simulink model "B5B3"  (R2015a)
settings: Solver=ode45  StartTime=0.0  StopTime=10.0  RelTol=1e-3
libraries: dspsrcs4 x4, commfilt2 x2, commchan3 x1, commsink2 x1, commutil2 x1, commrandsrc2 x1, dspstat3 x1
settings Model: Creator=Ekko  LastModifiedBy=Ekko

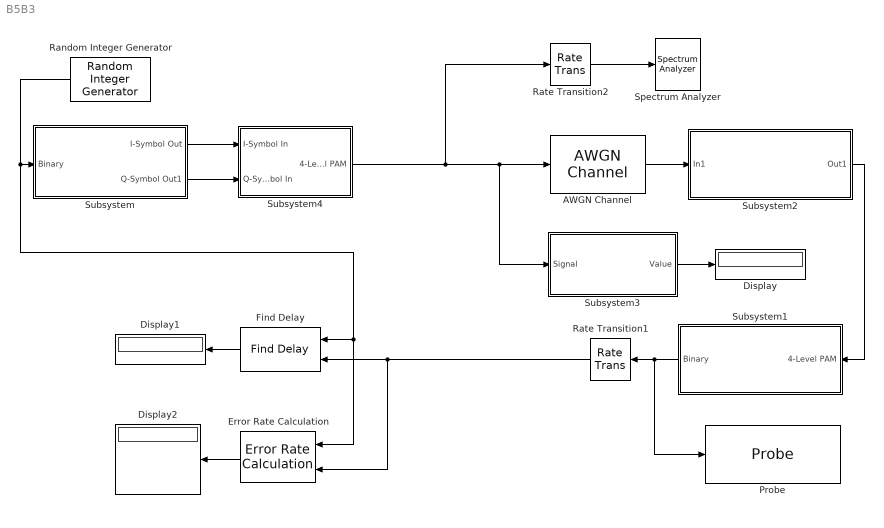
== system B5B3 ==
  AWGN Channel : commchan3/AWGN Channel  InputProcessing=Columns as channels (frame based)  seed=67  noiseMode="Signal to noise ratio  (Eb/No)"  EbNodB=8  EsNodB=10  SNRdB=10  bitsPerSym=1  Ps=1  Tsym=1  variance=1
  Display : Display
  Display1 : Display
  Display2 : Display
  Error Rate Calculation : commsink2/Error Rate Calculation  N=0  st_delay=0  cp_mode=Entire frame  subframe=[]  PMode=Port  WsName=ErrorVec  RsMode2=off  stop=off  numErr=100  maxBits=1e6
  Find Delay : commutil2/Find Delay  corrLength=200  chgSigOP=off  stopUpdate=off  numConstDelay=3
  Probe : Probe  ProbeWidth=off  ProbeComplexSignal=off  ProbeSignalDimensions=on
  Random Integer Generator : commrandsrc2/Random Integer Generator  mul=2  seed=37  Ts=1e-5  frameBased=off  sampPerFrame=1  orient=off  outDataType=double
  Rate Transition1 : RateTransition  OutPortSampleTime=1e-5
  Rate Transition2 : RateTransition  OutPortSampleTime=1e-5
  Spectrum Analyzer : SpectrumAnalyzer
  Subsystem : Subsystem
  Subsystem1 : Subsystem
  Subsystem2 : Subsystem
  Subsystem3 : Subsystem
  Subsystem4 : Subsystem
  wires:
  AWGN Channel/1 -> Subsystem2/1(In1)
  Subsystem1/1("Binary ") -> Probe/1, Rate Transition1/1
  Subsystem2/1(Out1) -> Subsystem1/1("4-Level PAM ")
  Subsystem3/1("Value ") -> Display/1
  Find Delay/1 -> Display1/1
  Error Rate Calculation/1 -> Display2/1
  Rate Transition1/1 -> Error Rate Calculation/2, Find Delay/2
  Subsystem/1(I-Symbol Out) -> Subsystem4/1(I-Symbol In)
  Subsystem/2(Q-Symbol Out1) -> Subsystem4/2(Q-Symbol In)
  Subsystem4/1(4-Level PAM) -> Rate Transition2/1, Subsystem3/1("Signal "), AWGN Channel/1
  Random Integer Generator/1 -> Find Delay/1, Error Rate Calculation/1, Subsystem/1("Binary ")
  Rate Transition2/1 -> Spectrum Analyzer/1

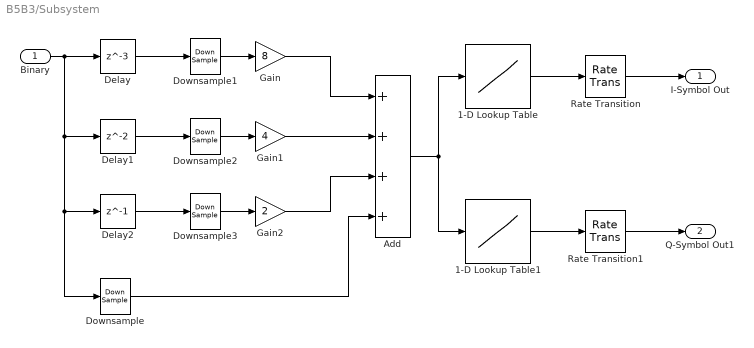
== system B5B3/Subsystem ==
  "Binary " : Inport
  1-D Lookup Table : Lookup_n-D  NumberOfTableDimensions=1  BreakpointsForDimension1=[0 1 2 3 4 5 6 7 8 9 10 11 12 13 14 15]  Table=[-1 -3 -1 -3 1 3 1 3 -1 -3 -1 -3 1 3 1 3]  InternalRulePriority=Speed  RndMeth=Simplest  InputSameDT=on
  1-D Lookup Table1 : Lookup_n-D  NumberOfTableDimensions=1  BreakpointsForDimension1=[0 1 2 3 4 5 6 7 8 9 10 11 12 13 14 15]  Table=[1 1 3 3 1 1 3 3 -1 -1 -3 -3 -1 -1 -3 -3]  InternalRulePriority=Speed  RndMeth=Simplest  InputSameDT=on
  Add : Sum  Inputs=4
  Delay : Delay  DelayLength=3
  Delay1 : Delay
  Delay2 : Delay  DelayLength=1
  Downsample{,1..3} (4 alike) : DownSample  N=4  RateOptions=Allow multirate processing
  Gain : Gain  Gain=8
  Gain1 : Gain  Gain=4
  Gain2 : Gain  Gain=2
  Rate Transition : RateTransition  OutPortSampleTime=1e-5
  Rate Transition1 : RateTransition  OutPortSampleTime=1e-5
  I-Symbol Out : Outport
  Q-Symbol Out1 : Outport  Port=2
  wires:
  "Binary "/1 -> Delay2/1, Downsample/1, Delay1/1, Delay/1
  Delay2/1 -> Downsample3/1
  Delay1/1 -> Downsample2/1
  Delay/1 -> Downsample1/1
  Downsample1/1 -> Gain/1
  Downsample2/1 -> Gain1/1
  Downsample3/1 -> Gain2/1
  Gain1/1 -> Add/2
  Gain/1 -> Add/1
  Gain2/1 -> Add/3
  Downsample/1 -> Add/4
  1-D Lookup Table1/1 -> Rate Transition1/1
  1-D Lookup Table/1 -> Rate Transition/1
  Add/1 -> 1-D Lookup Table1/1, 1-D Lookup Table/1
  Rate Transition1/1 -> Q-Symbol Out1/1
  Rate Transition/1 -> I-Symbol Out/1

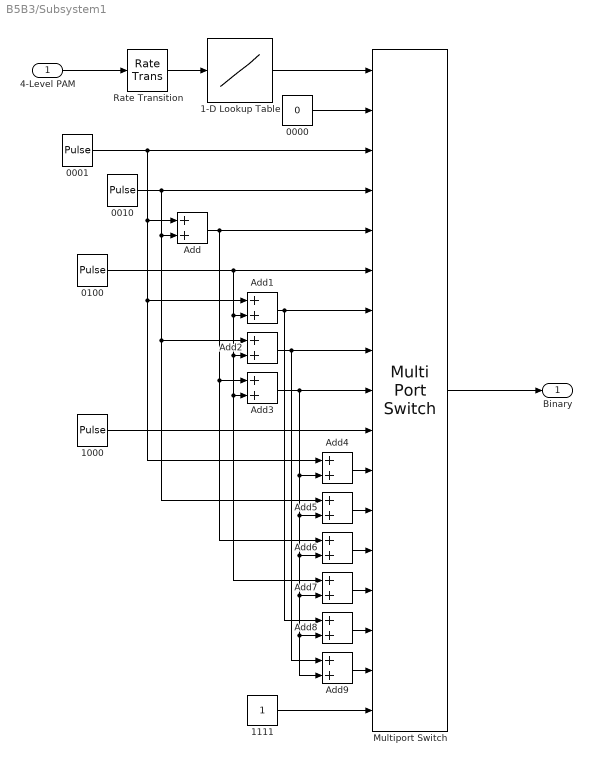
== system B5B3/Subsystem1 ==
  "4-Level PAM " : Inport
  0000 : Constant  Value=0  SampleTime=2e-5
  "0001 " : DiscretePulseGenerator  Amplitude=2  Period=50  PulseWidth=5  SampleTime=1e-5
  0010 : DiscretePulseGenerator  Amplitude=2  Period=10  PulseWidth=5  SampleTime=1e-5
  0100 : DiscretePulseGenerator  Amplitude=2  Period=10  PulseWidth=5  SampleTime=1e-5
  1-D Lookup Table : Lookup_n-D  NumberOfTableDimensions=1  BreakpointsForDimension1=[0 1]  Table=[-5 5]  InternalRulePriority=Speed  RndMeth=Simplest  InputSameDT=on
  1000 : DiscretePulseGenerator  Amplitude=2  Period=10  PulseWidth=5  SampleTime=1e-5
  "1111 " : Constant  SampleTime=2e-5
  Add{,1..9} (10 alike) : Sum
  Multiport Switch : MultiPortSwitch  Inputs=16  DiagnosticForDefault=None
  Rate Transition : RateTransition  OutPortSampleTime=1e-5
  "Binary " : Outport
  wires:
  Rate Transition/1 -> 1-D Lookup Table/1
  "4-Level PAM "/1 -> Rate Transition/1
  1-D Lookup Table/1 -> Multiport Switch/1
  0010/1 -> Add/2, Add2/1, Add5/1, Multiport Switch/4
  Multiport Switch/1 -> "Binary "/1
  "0001 "/1 -> Add/1, Add1/1, Add4/1, Multiport Switch/3
  0000/1 -> Multiport Switch/2
  "1111 "/1 -> Multiport Switch/17
  0100/1 -> Add1/2, Add2/2, Add3/2, Add7/1, Multiport Switch/6
  Add/1 -> Add6/1, Add3/1, Multiport Switch/5
  1000/1 -> Multiport Switch/10
  Add3/1 -> Add4/2, Add5/2, Add6/2, Add7/2, Add8/2, Add9/2, Multiport Switch/9
  Add2/1 -> Add9/1, Multiport Switch/8
  Add1/1 -> Add8/1, Multiport Switch/7
  Add4/1 -> Multiport Switch/11
  Add5/1 -> Multiport Switch/12
  Add6/1 -> Multiport Switch/13
  Add7/1 -> Multiport Switch/14
  Add8/1 -> Multiport Switch/15
  Add9/1 -> Multiport Switch/16

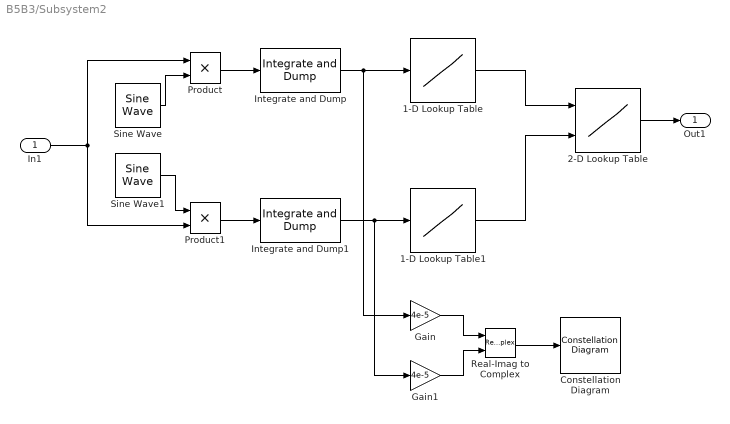
== system B5B3/Subsystem2 ==
  In1 : Inport
  1-D Lookup Table : Lookup_n-D  NumberOfTableDimensions=1  BreakpointsForDimension1=[0 1]  Table=[-5 5]  InternalRulePriority=Speed  RndMeth=Simplest  InputSameDT=on
  1-D Lookup Table1 : Lookup_n-D  NumberOfTableDimensions=1  BreakpointsForDimension1=[0 1]  Table=[-5 5]  InternalRulePriority=Speed  RndMeth=Simplest  InputSameDT=on
  2-D Lookup Table : Lookup_n-D  BreakpointsForDimension1=[1:3]  BreakpointsForDimension2=[1:3]  InternalRulePriority=Speed  RndMeth=Simplest  InputSameDT=on
  Constellation Diagram : ConstellationDiagram
  Gain : Gain  Gain=4e-5
  Gain1 : Gain  Gain=4e-5
  Integrate and Dump : commfilt2/Integrate and Dump  obssamples=8  offsetsamples=0  nodump=off  roundingMode=Floor  overflowMode=off
  Integrate and Dump1 : commfilt2/Integrate and Dump  obssamples=8  offsetsamples=0  nodump=off  roundingMode=Floor  overflowMode=off
  Product : Product
  Product1 : Product
  Real-Imag to Complex : RealImagToComplex
  Sine Wave : dspsrcs4/Sine Wave  Amplitude=1  Frequency=2000  Phase=0  SampleMode=Discrete  OutComplex=Real  CompMethod=Trigonometric fcn  TableSize=Speed  SampleTime=2e-5  SamplesPerFrame=1  ResetState=Restart at time zero  dataType=double  wordLen=16  udDataType=sfix(16)  fracBitsMode=Best precision  numFracBits=15  OutDataTypeStr=double  LastOutDataTypeStr=double
  Sine Wave1 : dspsrcs4/Sine Wave  Amplitude=1  Frequency=4000  Phase=0  SampleMode=Discrete  OutComplex=Real  CompMethod=Trigonometric fcn  TableSize=Speed  SampleTime=2e-5  SamplesPerFrame=1  ResetState=Restart at time zero  dataType=double  wordLen=16  udDataType=sfix(16)  fracBitsMode=Best precision  numFracBits=15  OutDataTypeStr=double  LastOutDataTypeStr=double
  Out1 : Outport
  wires:
  Product1/1 -> Integrate and Dump1/1
  Product/1 -> Integrate and Dump/1
  Sine Wave/1 -> Product/2
  In1/1 -> Product1/2, Product/1
  Sine Wave1/1 -> Product1/1
  Integrate and Dump/1 -> Gain/1, 1-D Lookup Table/1
  Integrate and Dump1/1 -> Gain1/1, 1-D Lookup Table1/1
  1-D Lookup Table/1 -> 2-D Lookup Table/1
  2-D Lookup Table/1 -> Out1/1
  Gain/1 -> Real-Imag to Complex/1
  Gain1/1 -> Real-Imag to Complex/2
  Real-Imag to Complex/1 -> Constellation Diagram/1
  1-D Lookup Table1/1 -> 2-D Lookup Table/2

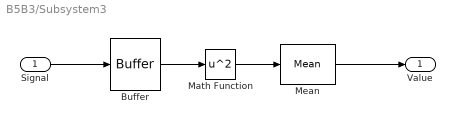
== system B5B3/Subsystem3 ==
  "Signal " : Inport
  Buffer : Buffer  TreatMby1Signals=One channel
  Math Function : Math  Operator=square  SaturateOnIntegerOverflow=on
  Mean : dspstat3/Mean  run=off  reset_popup=None  InputProcessing=Columns as channels (frame based)  directionMode=Each column  dimension=1  treatSBRowAsCol=off  roiEnable=off  roiType=Rectangles  roiPortion=Entire ROI  roiOutput=Individual statistics for each ROI  roiFlag=off  outputDataTypeStr=Inherit: Same as accumulator  outputLastDataTypeStr=Inherit: Same as accumulator  outputMin=[]  outputMax=[]  roundingMode=Floor  overflowMode=off
  "Value " : Outport
  wires:
  "Signal "/1 -> Buffer/1
  Mean/1 -> "Value "/1
  Math Function/1 -> Mean/1
  Buffer/1 -> Math Function/1

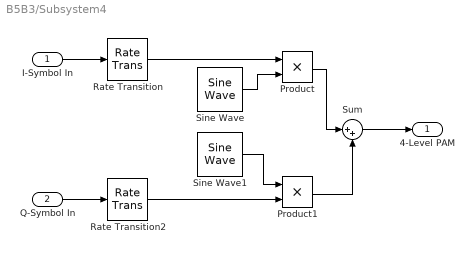
== system B5B3/Subsystem4 ==
  I-Symbol In : Inport
  Q-Symbol In : Inport  Port=2
  Product : Product
  Product1 : Product
  Rate Transition : RateTransition  OutPortSampleTime=1e-5
  Rate Transition2 : RateTransition  OutPortSampleTime=1e-5
  Sine Wave : dspsrcs4/Sine Wave  Amplitude=1  Frequency=100  Phase=0  SampleMode=Discrete  OutComplex=Real  CompMethod=Trigonometric fcn  TableSize=Speed  SampleTime=1/1000  SamplesPerFrame=1  ResetState=Restart at time zero  dataType=double  wordLen=16  udDataType=sfix(16)  fracBitsMode=Best precision  numFracBits=15  OutDataTypeStr=double  LastOutDataTypeStr=double
  Sine Wave1 : dspsrcs4/Sine Wave  Amplitude=1  Frequency=100  Phase=0  SampleMode=Discrete  OutComplex=Real  CompMethod=Trigonometric fcn  TableSize=Speed  SampleTime=1/1000  SamplesPerFrame=1  ResetState=Restart at time zero  dataType=double  wordLen=16  udDataType=sfix(16)  fracBitsMode=Best precision  numFracBits=15  OutDataTypeStr=double  LastOutDataTypeStr=double
  Sum : Sum  Inputs=|++
  4-Level PAM : Outport
  wires:
  Rate Transition2/1 -> Product1/2
  Product1/1 -> Sum/2
  Rate Transition/1 -> Product/1
  I-Symbol In/1 -> Rate Transition/1
  Sine Wave/1 -> Product/2
  Sum/1 -> 4-Level PAM/1
  Q-Symbol In/1 -> Rate Transition2/1
  Product/1 -> Sum/1
  Sine Wave1/1 -> Product1/1
